simulink model "sml_drivepose"  (R2016a)
settings: Solver=VariableStepAuto  StartTime=0.0  StopTime=20  RelTol=1e-3
libraries: simulink x1
settings Model: Creator=Duy Nam  LastModifiedBy=Duy Nam

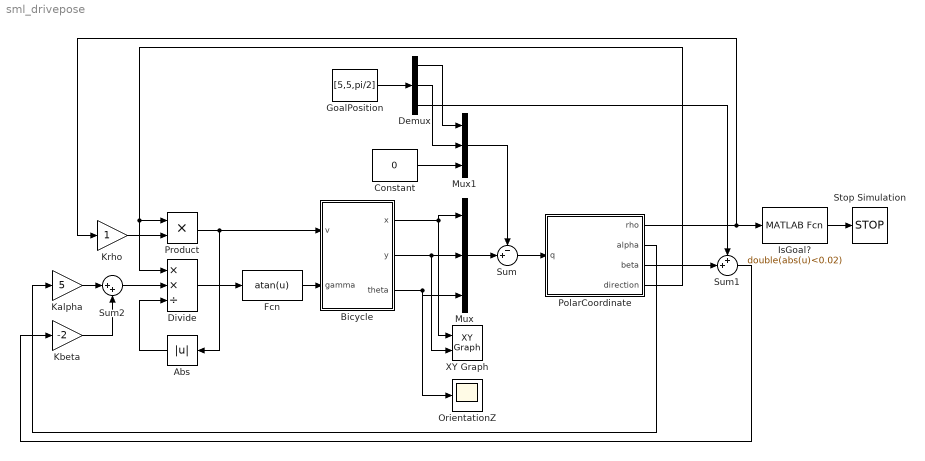
== system sml_drivepose ==
  Abs : Abs
  Bicycle : Subsystem
  Constant : Constant  Value=0
  Demux : Demux  Outputs=3
  Divide : Product  Inputs=**/
  Fcn : Fcn  Expr=atan(u)
  GoalPosition : Constant  Value=[5,5,pi/2]
  IsGoal? : MATLABFcn  MATLABFcn=double(abs(u)<0.02)  OutputSignalType=real
  Kalpha : Gain  Gain=5
  Kbeta : Gain  Gain=-2
  Krho : Gain
  Mux : Mux  Inputs=3
  Mux1 : Mux  Inputs=3
  OrientationZ : Scope
  PolarCoordinate : MATLAB Function  TreatAsAtomicUnit=on
  Product : Product
  Stop Simulation : Stop
  Sum : Sum  Inputs=-+|
  Sum1 : Sum  Inputs=++|
  Sum2 : Sum  Inputs=|++
  XY Graph : simulink/Sinks/XY Graph  xmin=0  xmax=10  ymin=0  ymax=10  st=-1
  wires:
  Fcn/1 -> Bicycle/2(gamma)
  Bicycle/1(x) -> XY Graph/1, Mux/1
  Bicycle/2(y) -> XY Graph/2, Mux/2
  Mux/1 -> Sum/2
  Bicycle/3(theta) -> OrientationZ/1, Mux/3
  Sum/1 -> PolarCoordinate/1(q)
  Mux1/1 -> Sum/1
  IsGoal?/1 -> Stop Simulation/1
  PolarCoordinate/1(rho) -> Krho/1, IsGoal?/1
  PolarCoordinate/3(beta) -> Sum1/2
  Product/1 -> Bicycle/1(v), Abs/1
  Krho/1 -> Product/2
  Abs/1 -> Divide/3
  Kalpha/1 -> Sum2/1
  Sum2/1 -> Divide/2
  Kbeta/1 -> Sum2/2
  Sum1/1 -> Kbeta/1
  PolarCoordinate/2(alpha) -> Kalpha/1
  Divide/1 -> Fcn/1
  PolarCoordinate/4(direction) -> Divide/1, Product/1
  GoalPosition/1 -> Demux/1
  Constant/1 -> Mux1/3
  Demux/3 -> Sum1/1
  Demux/2 -> Mux1/2
  Demux/1 -> Mux1/1

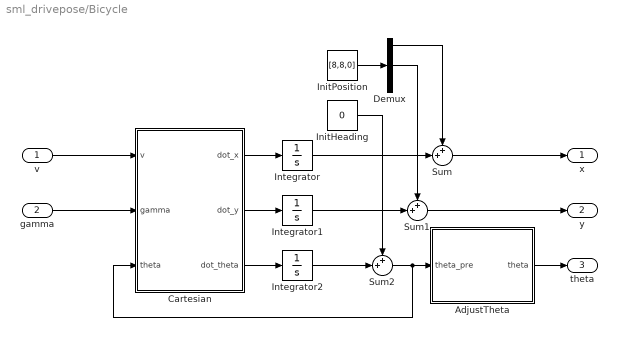
== system sml_drivepose/Bicycle ==
  v : Inport
  gamma : Inport  Port=2
  AdjustTheta : MATLAB Function  TreatAsAtomicUnit=on
  Cartesian : MATLAB Function  TreatAsAtomicUnit=on
  Demux : Demux  Outputs=3
  InitHeading : Constant  Value=0
  InitPosition : Constant  Value=[8,8,0]
  Integrator : Integrator
  Integrator1 : Integrator
  Integrator2 : Integrator
  Sum : Sum  Inputs=++|
  Sum1 : Sum  Inputs=++|
  Sum2 : Sum  Inputs=++|
  x : Outport
  y : Outport  Port=2
  theta : Outport  Port=3
  wires:
  Cartesian/1(dot_x) -> Integrator/1
  Integrator/1 -> Sum/2
  Cartesian/2(dot_y) -> Integrator1/1
  Integrator1/1 -> Sum1/2
  Cartesian/3(dot_theta) -> Integrator2/1
  AdjustTheta/1(theta) -> theta/1
  Sum2/1 -> Cartesian/3(theta), AdjustTheta/1(theta_pre)
  v/1 -> Cartesian/1(v)
  gamma/1 -> Cartesian/2(gamma)
  InitPosition/1 -> Demux/1
  Sum/1 -> x/1
  Demux/1 -> Sum/1
  Sum1/1 -> y/1
  Demux/2 -> Sum1/1
  Integrator2/1 -> Sum2/2
  InitHeading/1 -> Sum2/1

== matlab function sml_drivepose/Bicycle/AdjustTheta ==
  data: theta_pre input; theta output
function theta = AdjustTheta(theta_pre)
% ADJUSTTHETA Adjust the heading angle always between [-pi/2;pi/2]
%% INPUTS
% theta_pre = The heading angle before adjust
%% OUTPUTS
% theta = The heading angle after adjust
%% AdjustTheta
theta = theta_pre - 2*pi*floor((theta_pre + pi)/(2*pi));
end

== matlab function sml_drivepose/Bicycle/Cartesian ==
  data: dot_x output; dot_y output; v input; gamma input; theta input; dot_theta output
function [dot_x, dot_y, dot_theta] = Cartesian(v, gamma, theta)
% CARTESIAN Compute the velocity of robot in world frame
%% INPUTS
% v     = The velocity of the back wheel
% gamma = The steering wheel angle
% theta = The heading angle
%% OUTPUTS
% dot_x     = The velocity of robot in world frame x-axis
% dot_y     = The velocity of robot in world frame y-axis
% dot theta = The rate of change of heading
%% PARAMETERS
L = params_bicycle();
%% Cartesian
dot_x = v*cos(theta);
dot_y = v*sin(theta);
dot_theta = v/L*tan(gamma);
end

== matlab function sml_drivepose/PolarCoordinate ==
  data: q input; rho output; alpha output; beta output; direction output
function [rho, alpha, beta, direction] = PolarCoordinate(q)
% POLARCOORDINATE Convert to polar coordinate
%% INPUTS
% q = Error position of robot (Delta_x, Delta_y, theta)
%% OUTPUTS
% rho       = Distance from current position to the goal
% alpha     = The angle of the goal vector with respect to the vehicle frame
% beta      = The angle of the goal vector with respect to the world frame
% direction = The moving direction (forward = 1; backward = -1)
%% Get the position
Dx = q(1); Dy = q(2); theta = q(3);
%% Compute the output
rho = sqrt(Dx^2 + Dy^2);
beta = -atan2(-Dy, -Dx);
alpha = -theta - beta;
if abs(alpha) < pi/2
    direction = 1;
else
    direction = -1;
    beta = -atan2(Dy, Dx);
    alpha = -theta - beta;
end
end
